simulink model "Encoder_reader_simulink"  (R2025a)
settings: Solver=FixedStepAuto  StartTime=0.0  StopTime=inf  FixedStep=0.01  RelTol=1e-3  EnableMultiTasking=on
libraries: stm32f4xxblockslib x18, stm32g4xxblockslib x6
settings Model: STM32="{\"EncoderBlockForG4\":[{\"ID\":\"untitled:1\"},{\"ID\":\"Lab3_Encoder:1\"},{\"ID\":\"Encoder_reader_simulink:1\"},{\"ID\":\"Encoder_reader_simulink:65\"},{\"ID\":\"Encoder_reader_simulink:89\"},{\"ID\":\"Encoder_reader_simulink:257\"},{\"ID\":\"Encoder_reader_simulink:258\"},{\"ID\":\"Encoder_reader_simulink:259\"}],\"DigitalPortRead\":[{\"ID\":\"Encoder_reader_simulink:43\"},{\"ID\":\"Encoder_reader_simulink:60\"},{\"ID\":\"Encoder_reader_simulink:71\"},{\"ID\":\"Encoder_reader_simulink:72\"},{\"ID\":\"Encoder_reader_simulink:73\"},{\"ID\":\"Encoder_reader_simulink:74\"},{\"ID\":\"Encoder_reader_simulink:82\"},{\"ID\":\"Encoder_reader_simulink:83\"},{\"ID\":\"Encoder_reader_simulink:84\"},{\"ID\":\"Encoder_reader_simulink:236\"},{\"ID\":\"Encoder_reader_simulink:237\"},{\"ID\":\"Encoder_reader_simulink:238\"},{\"ID\":\"Encoder_reader_simulink:239\"},{\"ID\":\"Encoder_reader_simulink:240\"},{\"ID\":\"Encoder_reader_simulink:241\"},{\"ID\":\"Encoder_reader_simulink:242\"},{\"ID\":\"Encoder_reader_simulink:243\"},{\"ID\":\"Encoder_reader_simulink:235\"}]}"  Creator=User  LastModifiedBy=nitic
settings OptimizationCC: DefaultParameterBehavior=Inlined  EnhancedBackFolding=on  PassReuseOutputArgsAs=Individual arguments  ZeroExternalMemoryAtStartup=off  ZeroInternalMemoryAtStartup=off  MaxStackSize=512  OptimizeBlockOrder=speed  DifferentSizesBufferReuse=on  OptimizationCustomize=off  EfficientTunableParamExpr=on
settings DebuggingCC: ParameterTunabilityLossMsg=error
settings HardwareCC: ProdBitPerPointer=32.0  ProdBitPerSizeT=32.0  ProdBitPerPtrDiffT=32.0  ProdLargestAtomicInteger=Long  ProdLargestAtomicFloat=Double  ProdWordSize=32.0  ProdLongLongMode=on  ProdHWDeviceType=ARM Compatible->ARM Cortex-M
settings SFSimCC: MATLABDynamicMemAlloc=off
settings RTWCC: SystemTargetFile=ert.tlc  HardwareBoard=STM32G4xx Based  TemplateMakefile=ert_default_tmf  Toolchain=GNU Tools for ARM Embedded Processors  Description=Embedded Coder
settings CodeAppCC: ForceParamTrailComments=on  IgnoreCustomStorageClasses=off  OperatorAnnotations=on  SimulinkDataObjDesc=on  SFDataObjDesc=on  InsertBlockDesc=on
settings ERTTargetCC: ExtModeTransport=3.0  ExtModeStaticAllocSize=2048.0  TargetLangStandard=C99 (ISO)  CodeReplacementLibrary=ARM Cortex-M  SupportContinuousTime=on

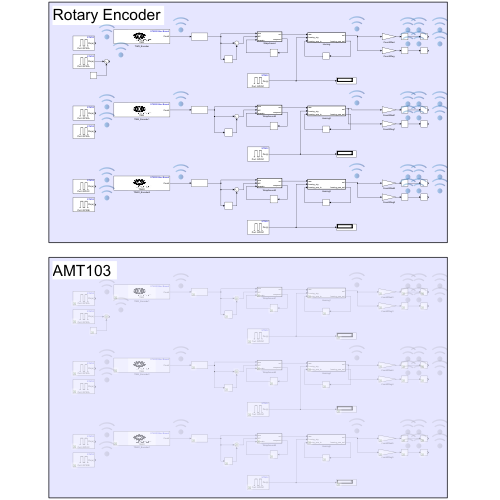
[thumbnail: Simulink's stored preview of the top-level diagram]
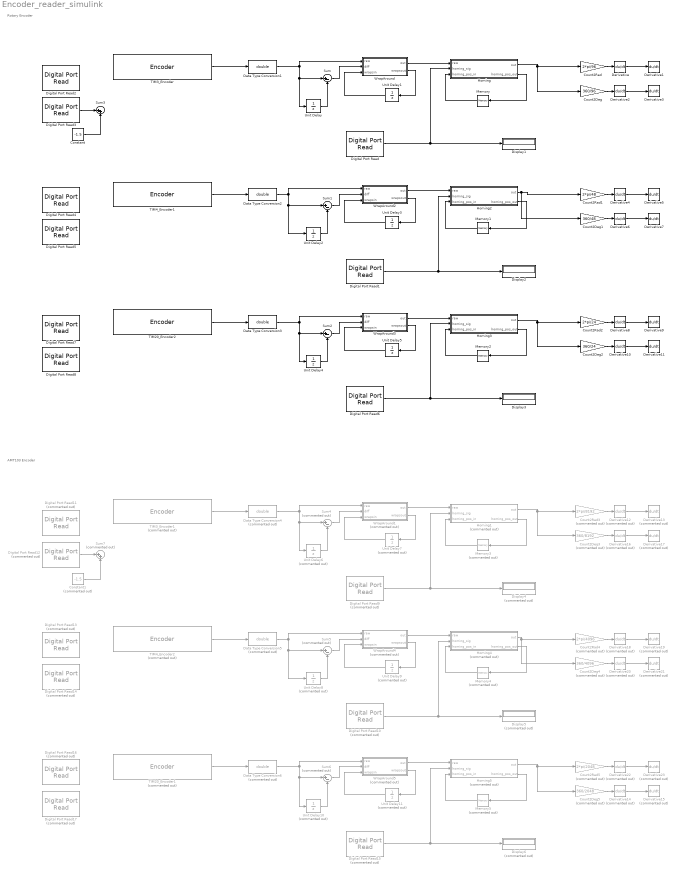
== system Encoder_reader_simulink ==
  note: Rotary Encoder
  note: AMT103 Encoder
  Constant : Constant  Value=-1.5
  Constant1 : Constant  Commented=on  Value=-1.5
  Count2Deg : Gain  Gain=360/96
  Count2Deg1 : Gain  Gain=360/48
  Count2Deg2 : Gain  Gain=360/24
  Count2Deg3 : Gain  Commented=on  Gain=360/8192
  Count2Deg4 : Gain  Commented=on  Gain=360/4096
  Count2Deg5 : Gain  Commented=on  Gain=360/2048
  Count2Rad : Gain  Gain=2*pi/96
  Count2Rad1 : Gain  Gain=2*pi/48
  Count2Rad2 : Gain  Gain=2*pi/24
  Count2Rad3 : Gain  Commented=on  Gain=2*pi/8192
  Count2Rad4 : Gain  Commented=on  Gain=2*pi/4096
  Count2Rad5 : Gain  Commented=on  Gain=2*pi/2048
  Data Type Conversion1 : DataTypeConversion  OutDataTypeStr=double  SaturateOnIntegerOverflow=off  RndMeth=Floor
  Data Type Conversion2 : DataTypeConversion  OutDataTypeStr=double  SaturateOnIntegerOverflow=off  RndMeth=Floor
  Data Type Conversion3 : DataTypeConversion  OutDataTypeStr=double  SaturateOnIntegerOverflow=off  RndMeth=Floor
  Data Type Conversion4 : DataTypeConversion  Commented=on  OutDataTypeStr=double  SaturateOnIntegerOverflow=off  RndMeth=Floor
  Data Type Conversion5 : DataTypeConversion  Commented=on  OutDataTypeStr=double  SaturateOnIntegerOverflow=off  RndMeth=Floor
  Data Type Conversion6 : DataTypeConversion  Commented=on  OutDataTypeStr=double  SaturateOnIntegerOverflow=off  RndMeth=Floor
  Derivative{,1..11} (12 alike) : Derivative
  Derivative{12..23} (12 alike) : Derivative  Commented=on
  Digital Port Read : stm32f4xxblockslib/Digital Port Read  PortName=GPIOC  PinNumber=[13]  ReadOperation=on  IOAsArray=on  SampleTime=-1  EnableSimPort=off  hoistedMaskSrc=ECSoC/ECSimCodegen/Digital Port Read
      settings: LibrarySourceBlock=stm32f2xxblockslib/Digital Port Read
  Digital Port Read1 : stm32f4xxblockslib/Digital Port Read  PortName=GPIOC  PinNumber=[13]  ReadOperation=on  IOAsArray=on  SampleTime=-1  EnableSimPort=off  hoistedMaskSrc=ECSoC/ECSimCodegen/Digital Port Read
      settings: LibrarySourceBlock=stm32f2xxblockslib/Digital Port Read
  Digital Port Read10 : stm32f4xxblockslib/Digital Port Read  Commented=on  PortName=GPIOC  PinNumber=[13]  ReadOperation=on  IOAsArray=on  SampleTime=-1  EnableSimPort=off  hoistedMaskSrc=ECSoC/ECSimCodegen/Digital Port Read
      settings: LibrarySourceBlock=stm32f2xxblockslib/Digital Port Read
  Digital Port Read11 : stm32f4xxblockslib/Digital Port Read  Commented=on  PortName=GPIOA  PinNumber=[4]  ReadOperation=on  IOAsArray=on  SampleTime=-1  EnableSimPort=off  hoistedMaskSrc=ECSoC/ECSimCodegen/Digital Port Read
      settings: LibrarySourceBlock=stm32f2xxblockslib/Digital Port Read
  Digital Port Read12 : stm32f4xxblockslib/Digital Port Read  Commented=on  PortName=GPIOA  PinNumber=[6]  ReadOperation=on  IOAsArray=on  SampleTime=-1  EnableSimPort=off  hoistedMaskSrc=ECSoC/ECSimCodegen/Digital Port Read
      settings: LibrarySourceBlock=stm32f2xxblockslib/Digital Port Read
  Digital Port Read13 : stm32f4xxblockslib/Digital Port Read  Commented=on  PortName=GPIOA  PinNumber=[11]  ReadOperation=on  IOAsArray=on  SampleTime=-1  EnableSimPort=off  hoistedMaskSrc=ECSoC/ECSimCodegen/Digital Port Read
      settings: LibrarySourceBlock=stm32f2xxblockslib/Digital Port Read
  Digital Port Read14 : stm32f4xxblockslib/Digital Port Read  Commented=on  PortName=GPIOA  PinNumber=[12]  ReadOperation=on  IOAsArray=on  SampleTime=-1  EnableSimPort=off  hoistedMaskSrc=ECSoC/ECSimCodegen/Digital Port Read
      settings: LibrarySourceBlock=stm32f2xxblockslib/Digital Port Read
  Digital Port Read15 : stm32f4xxblockslib/Digital Port Read  Commented=on  PortName=GPIOC  PinNumber=[13]  ReadOperation=on  IOAsArray=on  SampleTime=-1  EnableSimPort=off  hoistedMaskSrc=ECSoC/ECSimCodegen/Digital Port Read
      settings: LibrarySourceBlock=stm32f2xxblockslib/Digital Port Read
  Digital Port Read16 : stm32f4xxblockslib/Digital Port Read  Commented=on  PortName=GPIOC  PinNumber=[3]  ReadOperation=on  IOAsArray=on  SampleTime=-1  EnableSimPort=off  hoistedMaskSrc=ECSoC/ECSimCodegen/Digital Port Read
      settings: LibrarySourceBlock=stm32f2xxblockslib/Digital Port Read
  Digital Port Read17 : stm32f4xxblockslib/Digital Port Read  Commented=on  PortName=GPIOB  PinNumber=[2]  ReadOperation=on  IOAsArray=on  SampleTime=-1  EnableSimPort=off  hoistedMaskSrc=ECSoC/ECSimCodegen/Digital Port Read
      settings: LibrarySourceBlock=stm32f2xxblockslib/Digital Port Read
  Digital Port Read2 : stm32f4xxblockslib/Digital Port Read  PortName=GPIOA  PinNumber=[4]  ReadOperation=on  IOAsArray=on  SampleTime=-1  EnableSimPort=off  hoistedMaskSrc=ECSoC/ECSimCodegen/Digital Port Read
      settings: LibrarySourceBlock=stm32f2xxblockslib/Digital Port Read
  Digital Port Read3 : stm32f4xxblockslib/Digital Port Read  PortName=GPIOA  PinNumber=[6]  ReadOperation=on  IOAsArray=on  SampleTime=-1  EnableSimPort=off  hoistedMaskSrc=ECSoC/ECSimCodegen/Digital Port Read
      settings: LibrarySourceBlock=stm32f2xxblockslib/Digital Port Read
  Digital Port Read4 : stm32f4xxblockslib/Digital Port Read  PortName=GPIOA  PinNumber=[11]  ReadOperation=on  IOAsArray=on  SampleTime=-1  EnableSimPort=off  hoistedMaskSrc=ECSoC/ECSimCodegen/Digital Port Read
      settings: LibrarySourceBlock=stm32f2xxblockslib/Digital Port Read
  Digital Port Read5 : stm32f4xxblockslib/Digital Port Read  PortName=GPIOA  PinNumber=[12]  ReadOperation=on  IOAsArray=on  SampleTime=-1  EnableSimPort=off  hoistedMaskSrc=ECSoC/ECSimCodegen/Digital Port Read
      settings: LibrarySourceBlock=stm32f2xxblockslib/Digital Port Read
  Digital Port Read6 : stm32f4xxblockslib/Digital Port Read  PortName=GPIOC  PinNumber=[13]  ReadOperation=on  IOAsArray=on  SampleTime=-1  EnableSimPort=off  hoistedMaskSrc=ECSoC/ECSimCodegen/Digital Port Read
      settings: LibrarySourceBlock=stm32f2xxblockslib/Digital Port Read
  Digital Port Read7 : stm32f4xxblockslib/Digital Port Read  PortName=GPIOC  PinNumber=[3]  ReadOperation=on  IOAsArray=on  SampleTime=-1  EnableSimPort=off  hoistedMaskSrc=ECSoC/ECSimCodegen/Digital Port Read
      settings: LibrarySourceBlock=stm32f2xxblockslib/Digital Port Read
  Digital Port Read8 : stm32f4xxblockslib/Digital Port Read  PortName=GPIOB  PinNumber=[2]  ReadOperation=on  IOAsArray=on  SampleTime=-1  EnableSimPort=off  hoistedMaskSrc=ECSoC/ECSimCodegen/Digital Port Read
      settings: LibrarySourceBlock=stm32f2xxblockslib/Digital Port Read
  Digital Port Read9 : stm32f4xxblockslib/Digital Port Read  Commented=on  PortName=GPIOC  PinNumber=[13]  ReadOperation=on  IOAsArray=on  SampleTime=-1  EnableSimPort=off  hoistedMaskSrc=ECSoC/ECSimCodegen/Digital Port Read
      settings: LibrarySourceBlock=stm32f2xxblockslib/Digital Port Read
  Display1 : Display
  Display2 : Display
  Display3 : Display
  Display4 : Display  Commented=on
  Display5 : Display  Commented=on
  Display6 : Display  Commented=on
  Homing : MATLAB Function  TreatAsAtomicUnit=on
  Homing1 : MATLAB Function  Commented=on  TreatAsAtomicUnit=on
  Homing2 : MATLAB Function  TreatAsAtomicUnit=on
  Homing3 : MATLAB Function  TreatAsAtomicUnit=on
  Homing4 : MATLAB Function  Commented=on  TreatAsAtomicUnit=on
  Homing5 : MATLAB Function  Commented=on  TreatAsAtomicUnit=on
  Memory : Memory
  Memory1 : Memory
  Memory2 : Memory
  Memory3 : Memory  Commented=on
  Memory4 : Memory  Commented=on
  Memory5 : Memory  Commented=on
  Sum : Sum  Inputs=|+-
  Sum1 : Sum  Inputs=|+-
  Sum2 : Sum  Inputs=|+-
  Sum3 : Sum  Inputs=|++
  Sum4 : Sum  Commented=on  Inputs=|+-
  Sum5 : Sum  Commented=on  Inputs=|+-
  Sum6 : Sum  Commented=on  Inputs=|+-
  Sum7 : Sum  Commented=on  Inputs=|++
  TIM20_Encoder1 : stm32g4xxblockslib/Encoder  Commented=on  TimerModule=TIM20  EnableResetInput=off  OutputCountAfterFirstIndex=off  OutputValidIndex=off  OutputDirection=off  OutputStatus=off  SampleTime=-1
  TIM20_Encoder2 : stm32g4xxblockslib/Encoder  TimerModule=TIM20  EnableResetInput=off  OutputCountAfterFirstIndex=off  OutputValidIndex=off  OutputDirection=off  OutputStatus=off  SampleTime=-1
  TIM3_Encoder : stm32g4xxblockslib/Encoder  TimerModule=TIM3  EnableResetInput=off  OutputCountAfterFirstIndex=off  OutputValidIndex=off  OutputDirection=off  OutputStatus=off  SampleTime=-1
  TIM3_Encoder1 : stm32g4xxblockslib/Encoder  Commented=on  TimerModule=TIM3  EnableResetInput=off  OutputCountAfterFirstIndex=off  OutputValidIndex=off  OutputDirection=off  OutputStatus=off  SampleTime=-1
  TIM4_Encoder1 : stm32g4xxblockslib/Encoder  TimerModule=TIM4  EnableResetInput=off  OutputCountAfterFirstIndex=off  OutputValidIndex=off  OutputDirection=off  OutputStatus=off  SampleTime=-1
  TIM4_Encoder2 : stm32g4xxblockslib/Encoder  Commented=on  TimerModule=TIM4  EnableResetInput=off  OutputCountAfterFirstIndex=off  OutputValidIndex=off  OutputDirection=off  OutputStatus=off  SampleTime=-1
  Unit Delay{,1..5} (6 alike) : UnitDelay  SampleTime=-1  HasFrameUpgradeWarning=on
  Unit Delay{6..11} (6 alike) : UnitDelay  Commented=on  SampleTime=-1  HasFrameUpgradeWarning=on
  WrapAround : MATLAB Function  TreatAsAtomicUnit=on
  WrapAround1 : MATLAB Function  Commented=on  TreatAsAtomicUnit=on
  WrapAround2 : MATLAB Function  TreatAsAtomicUnit=on
  WrapAround3 : MATLAB Function  TreatAsAtomicUnit=on
  WrapAround4 : MATLAB Function  Commented=on  TreatAsAtomicUnit=on
  WrapAround5 : MATLAB Function  Commented=on  TreatAsAtomicUnit=on
  wires:
  TIM3_Encoder/1 -> Data Type Conversion1/1
  Data Type Conversion1/1 -> WrapAround/1(raw), Unit Delay/1, Sum/1
  Derivative/1 -> Derivative1/1
  WrapAround/1(out) -> Homing/1(raw)
  Count2Rad/1 -> Derivative/1
  Count2Deg/1 -> Derivative2/1
  Derivative2/1 -> Derivative3/1
  Unit Delay/1 -> Sum/2
  Sum/1 -> WrapAround/2(diff)
  WrapAround/2(wrapsout) -> Unit Delay1/1
  Unit Delay1/1 -> WrapAround/3(wrapsin)
  Digital Port Read/1 -> Homing/2(homing_sig), Display1/1
  Homing/2(homing_pos_out) -> Memory/1
  Memory/1 -> Homing/3(homing_pos_in)
  Homing/1(out) -> Count2Deg/1, Count2Rad/1
  Homing2/1(out) -> Count2Deg1/1, Count2Rad1/1
  Homing2/2(homing_pos_out) -> Memory1/1
  Digital Port Read1/1 -> Homing2/2(homing_sig), Display2/1
  Memory1/1 -> Homing2/3(homing_pos_in)
  Unit Delay3/1 -> WrapAround2/3(wrapsin)
  Data Type Conversion2/1 -> Unit Delay2/1, Sum1/1, WrapAround2/1(raw)
  Derivative4/1 -> Derivative5/1
  Count2Deg1/1 -> Derivative6/1
  Sum1/1 -> WrapAround2/2(diff)
  WrapAround2/2(wrapsout) -> Unit Delay3/1
  TIM4_Encoder1/1 -> Data Type Conversion2/1
  WrapAround2/1(out) -> Homing2/1(raw)
  Derivative6/1 -> Derivative7/1
  Count2Rad1/1 -> Derivative4/1
  Unit Delay2/1 -> Sum1/2
  Homing3/1(out) -> Count2Deg2/1, Count2Rad2/1
  Unit Delay4/1 -> Sum2/2
  Derivative10/1 -> Derivative11/1
  Count2Rad2/1 -> Derivative8/1
  TIM20_Encoder2/1 -> Data Type Conversion3/1
  WrapAround3/2(wrapsout) -> Unit Delay5/1
  Count2Deg2/1 -> Derivative10/1
  Sum2/1 -> WrapAround3/2(diff)
  Data Type Conversion3/1 -> WrapAround3/1(raw), Unit Delay4/1, Sum2/1
  Derivative8/1 -> Derivative9/1
  WrapAround3/1(out) -> Homing3/1(raw)
  Memory2/1 -> Homing3/3(homing_pos_in)
  Unit Delay5/1 -> WrapAround3/3(wrapsin)
  Homing3/2(homing_pos_out) -> Memory2/1
  Digital Port Read6/1 -> Homing3/2(homing_sig), Display3/1
  Digital Port Read3/1 -> Sum3/1
  Constant/1 -> Sum3/2
  Count2Rad4/1 -> Derivative18/1
  Constant1/1 -> Sum7/2
  Derivative22/1 -> Derivative23/1
  Count2Rad3/1 -> Derivative12/1
  WrapAround5/1(out) -> Homing5/1(raw)
  Digital Port Read10/1 -> Homing4/2(homing_sig), Display5/1
  Count2Deg5/1 -> Derivative14/1
  Memory3/1 -> Homing1/3(homing_pos_in)
  Unit Delay10/1 -> Sum6/2
  TIM4_Encoder2/1 -> Data Type Conversion5/1
  Memory5/1 -> Homing5/3(homing_pos_in)
  Count2Deg4/1 -> Derivative20/1
  Unit Delay9/1 -> WrapAround4/3(wrapsin)
  Data Type Conversion6/1 -> WrapAround5/1(raw), Unit Delay10/1, Sum6/1
  Unit Delay6/1 -> Sum4/2
  Count2Deg3/1 -> Derivative16/1
  TIM3_Encoder1/1 -> Data Type Conversion4/1
  Derivative14/1 -> Derivative15/1
  Derivative20/1 -> Derivative21/1
  Derivative18/1 -> Derivative19/1
  WrapAround4/1(out) -> Homing4/1(raw)
  Digital Port Read15/1 -> Homing5/2(homing_sig), Display6/1
  Data Type Conversion4/1 -> WrapAround1/1(raw), Unit Delay6/1, Sum4/1
  Homing1/2(homing_pos_out) -> Memory3/1
  Homing5/2(homing_pos_out) -> Memory5/1
  Homing4/1(out) -> Count2Deg4/1, Count2Rad4/1
  Sum4/1 -> WrapAround1/2(diff)
  Homing5/1(out) -> Count2Deg5/1, Count2Rad5/1
  WrapAround5/2(wrapsout) -> Unit Delay11/1
  Digital Port Read9/1 -> Homing1/2(homing_sig), Display4/1
  Digital Port Read12/1 -> Sum7/1
  Derivative12/1 -> Derivative13/1
  Derivative16/1 -> Derivative17/1
  WrapAround1/2(wrapsout) -> Unit Delay7/1
  Unit Delay11/1 -> WrapAround5/3(wrapsin)
  Count2Rad5/1 -> Derivative22/1
  WrapAround4/2(wrapsout) -> Unit Delay9/1
  WrapAround1/1(out) -> Homing1/1(raw)
  Sum6/1 -> WrapAround5/2(diff)
  Homing4/2(homing_pos_out) -> Memory4/1
  TIM20_Encoder1/1 -> Data Type Conversion6/1
  Unit Delay8/1 -> Sum5/2
  Memory4/1 -> Homing4/3(homing_pos_in)
  Homing1/1(out) -> Count2Deg3/1, Count2Rad3/1
  Unit Delay7/1 -> WrapAround1/3(wrapsin)
  Data Type Conversion5/1 -> Unit Delay8/1, Sum5/1, WrapAround4/1(raw)
  Sum5/1 -> WrapAround4/2(diff)

== matlab function Encoder_reader_simulink/Homing ==
  data: raw input; out output; homing_sig input; homing_pos_in input; homing_pos_out output
function [out,homing_pos_out]= fcn(raw, homing_sig,homing_pos_in)

if homing_sig == 1
    homing_pos_out = raw;
    out = 0;
else
    homing_pos_out = homing_pos_in;
    out = raw - homing_pos_in;
end

== matlab function Encoder_reader_simulink/WrapAround1 ==
  data: raw input; out output; diff input; wrapsout output; wrapsin input
function [out,wrapsout] = fcn(raw, diff, wrapsin)

capcity = 61439;

if diff >= capcity/2 %max
    out = -raw+(wrapsin+1)*capcity;
    wrapsout = wrapsin-1;
elseif diff <= -capcity/2 %min
    out = raw+(wrapsin+1)*capcity;
    wrapsout = wrapsin+1;
else
    out = raw+wrapsin*capcity;
    wrapsout = wrapsin;

end

== matlab function Encoder_reader_simulink/WrapAround4 ==
  data: raw input; out output; diff input; wrapsout output; wrapsin input
function [out,wrapsout] = fcn(raw, diff, wrapsin)

capcity = 61439;

if diff >= capcity/2 %max
    out = -raw+(wrapsin+1)*capcity;
    wrapsout = wrapsin-1;
elseif diff <= -capcity/2 %min
    out = raw+(wrapsin+1)*capcity;
    wrapsout = wrapsin+1;
else
    out = raw+wrapsin*capcity;
    wrapsout = wrapsin;

end

== matlab function Encoder_reader_simulink/WrapAround5 ==
  data: raw input; out output; diff input; wrapsout output; wrapsin input
function [out,wrapsout] = fcn(raw, diff, wrapsin)

capcity = 61439;

if diff >= capcity/2 %max
    out = -raw+(wrapsin+1)*capcity;
    wrapsout = wrapsin-1;
elseif diff <= -capcity/2 %min
    out = raw+(wrapsin+1)*capcity;
    wrapsout = wrapsin+1;
else
    out = raw+wrapsin*capcity;
    wrapsout = wrapsin;

end

== matlab function Encoder_reader_simulink/WrapAround ==
  data: raw input; out output; diff input; wrapsout output; wrapsin input
function [out,wrapsout] = fcn(raw, diff, wrapsin)

capcity = 61439;

if diff >= capcity/2 %max
    out = -raw+(wrapsin+1)*capcity;
    wrapsout = wrapsin-1;
elseif diff <= -capcity/2 %min
    out = raw+(wrapsin+1)*capcity;
    wrapsout = wrapsin+1;
else
    out = raw+wrapsin*capcity;
    wrapsout = wrapsin;

end

== matlab function Encoder_reader_simulink/Homing2 ==
  data: raw input; out output; homing_sig input; homing_pos_in input; homing_pos_out output
function [out,homing_pos_out]= fcn(raw, homing_sig,homing_pos_in)

if homing_sig == 1
    homing_pos_out = raw;
    out = 0;
else
    homing_pos_out = homing_pos_in;
    out = raw - homing_pos_in;
end

== matlab function Encoder_reader_simulink/WrapAround2 ==
  data: raw input; out output; diff input; wrapsout output; wrapsin input
function [out,wrapsout] = fcn(raw, diff, wrapsin)

capcity = 61439;

if diff >= capcity/2 %max
    out = -raw+(wrapsin+1)*capcity;
    wrapsout = wrapsin-1;
elseif diff <= -capcity/2 %min
    out = raw+(wrapsin+1)*capcity;
    wrapsout = wrapsin+1;
else
    out = raw+wrapsin*capcity;
    wrapsout = wrapsin;

end

== matlab function Encoder_reader_simulink/Homing3 ==
  data: raw input; out output; homing_sig input; homing_pos_in input; homing_pos_out output
function [out,homing_pos_out]= fcn(raw, homing_sig,homing_pos_in)

if homing_sig == 1
    homing_pos_out = raw;
    out = 0;
else
    homing_pos_out = homing_pos_in;
    out = raw - homing_pos_in;
end

== matlab function Encoder_reader_simulink/WrapAround3 ==
  data: raw input; out output; diff input; wrapsout output; wrapsin input
function [out,wrapsout] = fcn(raw, diff, wrapsin)

capcity = 61439;

if diff >= capcity/2 %max
    out = -raw+(wrapsin+1)*capcity;
    wrapsout = wrapsin-1;
elseif diff <= -capcity/2 %min
    out = raw+(wrapsin+1)*capcity;
    wrapsout = wrapsin+1;
else
    out = raw+wrapsin*capcity;
    wrapsout = wrapsin;

end

== matlab function Encoder_reader_simulink/Homing1 ==
  data: raw input; out output; homing_sig input; homing_pos_in input; homing_pos_out output
function [out,homing_pos_out]= fcn(raw, homing_sig,homing_pos_in)

if homing_sig == 1
    homing_pos_out = raw;
    out = 0;
else
    homing_pos_out = homing_pos_in;
    out = raw - homing_pos_in;
end

== matlab function Encoder_reader_simulink/Homing4 ==
  data: raw input; out output; homing_sig input; homing_pos_in input; homing_pos_out output
function [out,homing_pos_out]= fcn(raw, homing_sig,homing_pos_in)

if homing_sig == 1
    homing_pos_out = raw;
    out = 0;
else
    homing_pos_out = homing_pos_in;
    out = raw - homing_pos_in;
end

== matlab function Encoder_reader_simulink/Homing5 ==
  data: raw input; out output; homing_sig input; homing_pos_in input; homing_pos_out output
function [out,homing_pos_out]= fcn(raw, homing_sig,homing_pos_in)

if homing_sig == 1
    homing_pos_out = raw;
    out = 0;
else
    homing_pos_out = homing_pos_in;
    out = raw - homing_pos_in;
end
